simulink model "dynmodel_KUKA"  (R2016a)
settings: Solver=VariableStepAuto  StartTime=0.0  StopTime=10.0  MaxStep=1e-3  RelTol=1e-3
values from neighbouring files (symbols this model uses):
  th_DHM = -th_KUKA + offset    [dynamique_youbot.m]
libraries: simulink x1, dspmtrx3 x1
settings Model: Creator=Makarov_Mar  LastModifiedBy=Makarov_Mar

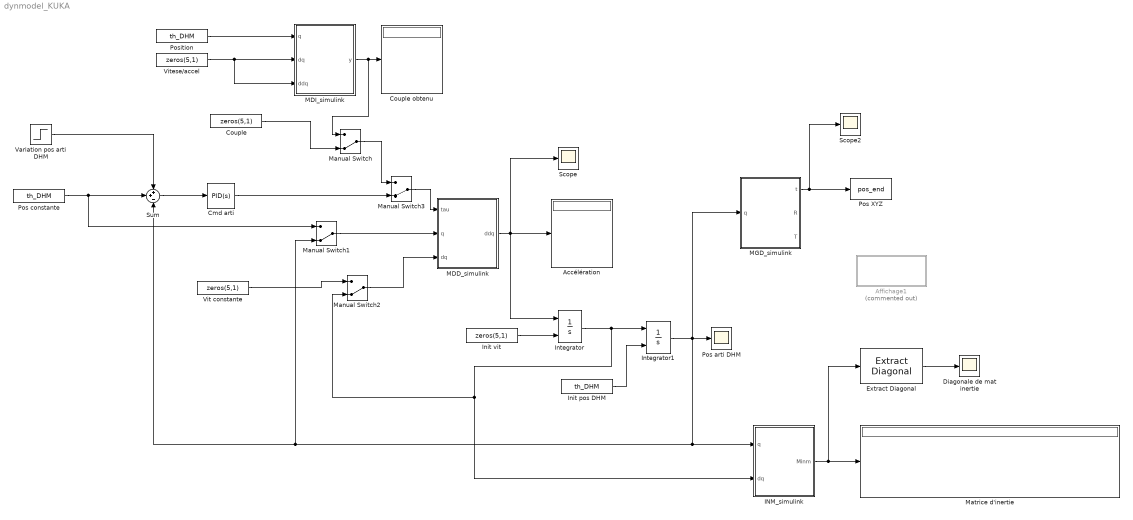
== system dynmodel_KUKA ==
  Accélération : Display
  Affichage1 : Subsystem  Commented=on  StopFcn=|
      | tps_sim =  pos_end.time;
      | PendX = pos_end.signals.values(:,1);
      | PendY = pos_end.signals.values(:,2);
      | PendZ = pos_end.signals.values(:,3);
      | 
      | figure(20)
      | for k = 1:70:length(tps_sim)
      |   figure(20)
      |   plot3(0,0,0,'r.','markersize',20); grid on; hold on
      |   axis([-0.7 0.7 -0.7 0.7 -1 +1])
      |   plot3(PendX(k),PendY(k),PendZ(k),'b.','markersize',10)
      |   xlabel('xB'); ylabel('yB'); zlabel('zB')
      |   title('xend : vert, yend : cyan, zend : rouge') 
      |   pause(0.1)
      | end
  Cmd arti : simulink/Continuous/PID Controller  Controller=PID  TimeDomain=Continuous-time  SampleTime=-1  IntegratorMethod=Forward Euler  FilterMethod=Forward Euler  Form=Parallel  UseFilter=on  ControllerParametersSource=internal  P=Kp.'  I=zeros(5,1)  D=Kd.'  N=10  InitialConditionSource=internal  InitialConditionForIntegrator=0  InitialConditionForFilter=0  ExternalReset=none  LimitOutput=off  UpperSaturationLimit=inf  LowerSaturationLimit=-inf  LinearizeAsGain=on  AntiWindupMode=none  Kb=1  TrackingMode=off  Kt=1  PParamMin=[]  PParamMax=[]  IParamMin=[]  IParamMax=[]  DParamMin=[]  DParamMax=[]  NParamMin=[]  NParamMax=[]  KbParamMin=[]  KbParamMax=[]  KtParamMin=[]  KtParamMax=[]  POutMin=[]  POutMax=[]  IOutMin=[]  IOutMax=[]  DOutMin=[]  DOutMax=[]  NOutMin=[]  NOutMax=[]  KbOutMin=[]  KbOutMax=[]  KtOutMin=[]  KtOutMax=[]  IntegratorOutMin=[]  IntegratorOutMax=[]  FilterOutMin=[]  FilterOutMax=[]  SumOutMin=[]  SumOutMax=[]  SumI1OutMin=[]  SumI1OutMax=[]  SumI2OutMin=[]  SumI2OutMax=[]  SumI3OutMin=[]  SumI3OutMax=[]  SumDOutMin=[]  SumDOutMax=[]  SaturationOutMin=[]  SaturationOutMax=[]  IntegratorContinuousStateAttributes=''  IntegratorStateMustResolveToSignalObject=off  IntegratorRTWStateStorageClass=Auto  FilterContinuousStateAttributes=''  FilterStateMustResolveToSignalObject=off  FilterRTWStateStorageClass=Auto  DifferentiatorICPrevScaledInput=0  DifferentiatorOutMin=[]  DifferentiatorOutMax=[]
  Couple : Constant  Value=zeros(5,1)  VectorParams1D=off
  Couple obtenu : Display
  Diagonale de mat inertie : Scope
  Extract Diagonal : dspmtrx3/Extract Diagonal
  INM_simulink : MATLAB Function  TreatAsAtomicUnit=on
  Init pos DHM : Constant  Value=th_DHM  VectorParams1D=off
  Init vit : Constant  Value=zeros(5,1)  VectorParams1D=off
  Integrator : Integrator  InitialConditionSource=external
  Integrator1 : Integrator  InitialConditionSource=external
  MDD_simulink : MATLAB Function  TreatAsAtomicUnit=on
  MDI_simulink : MATLAB Function  TreatAsAtomicUnit=on
  MGD_simulink : MATLAB Function  TreatAsAtomicUnit=on
  Manual Switch{,1..3} (4 alike) : ManualSwitch  CurrentSetting=0
  Matrice d'inertie : Display
  Pos XYZ : ToWorkspace  VariableName=pos_end  SaveFormat=Structure With Time  SampleTime=-1
  Pos arti DHM : Scope
  Pos constante : Constant  Value=th_DHM  VectorParams1D=off
  Position : Constant  Value=th_DHM  VectorParams1D=off
  Scope : Scope
  Scope2 : Scope
  Sum : Sum  Inputs=++-
  Variation pos arti DHM : Step  After=[0 pi/2 0 0 0]  SampleTime=0
  Vit constante : Constant  Value=zeros(5,1)  VectorParams1D=off
  Vitese/accel : Constant  Value=zeros(5,1)  VectorParams1D=off
  wires:
  Vitese/accel/1 -> MDI_simulink/2(dq), MDI_simulink/3(ddq)
  Position/1 -> MDI_simulink/1(q)
  MDI_simulink/1(y) -> Manual Switch/1, Couple obtenu/1
  MDD_simulink/1(ddq) -> Integrator/1, Scope/1, Accélération/1
  Couple/1 -> Manual Switch/2
  Integrator/1 -> INM_simulink/2(dq), Manual Switch2/2, Integrator1/1
  Init vit/1 -> Integrator/2
  Init pos DHM/1 -> Integrator1/2
  Pos constante/1 -> Sum/2, Manual Switch1/1
  Manual Switch1/1 -> MDD_simulink/2(q)
  Vit constante/1 -> Manual Switch2/1
  Manual Switch2/1 -> MDD_simulink/3(dq)
  Integrator1/1 -> MGD_simulink/1(q), Sum/3, Manual Switch1/2, INM_simulink/1(q), Pos arti DHM/1
  MGD_simulink/1(t) -> Scope2/1, Pos XYZ/1
  INM_simulink/1(Minm) -> Extract Diagonal/1, Matrice d'inertie/1
  Extract Diagonal/1 -> Diagonale de mat inertie/1
  Manual Switch/1 -> Manual Switch3/1
  Manual Switch3/1 -> MDD_simulink/1(tau)
  Cmd arti/1 -> Manual Switch3/2
  Sum/1 -> Cmd arti/1
  Variation pos arti DHM/1 -> Sum/1

== system dynmodel_KUKA/Affichage1 ==

== matlab function dynmodel_KUKA/MDD_simulink ==
  data: tau input; q input; dq input; ddq output size=5; param parameter
function ddq = fcn(tau,q,dq, param)

th1 = q(1);
th2 = q(2);
th3 = q(3);
th4 = q(4);
th5 = q(5);

QP1 = dq(1);
QP2 = dq(2);
QP3 = dq(3);
QP4 = dq(4);
QP5 = dq(5);

GAM1 =tau(1);
GAM2 =tau(2);
GAM3 =tau(3);
GAM4 =tau(4);
GAM5 = tau(5);

% introduction des paramètres
GZ=param.GZ;
XXR2=param.XXR2;
XXR3=param.XXR3;
XXR4=param.XXR4;
XXR5=param.XXR5;
XY2=param.XY2;
XY3=param.XY3;
XY4=param.XY4;
XY5=param.XY5;
XZR2=param.XZR2;
XZR3=param.XZR3;
XZ4=param.XZ4;
XZ5=param.XZ5;
YZ2=param.YZ2;
YZ3=param.YZ3;
YZ4=param.YZ4;
YZ5=param.YZ5;
ZZR1=param.ZZR1;
ZZR2=param.ZZR2;
ZZR3=param.ZZR3;
ZZR4=param.ZZR4;
ZZ5=param.ZZ5;
MXR2=param.MXR2;
MXR3=param.MXR3;
MX4=param.MX4;
MX5=param.MX5;
MY2=param.MY2;
MY3=param.MY3;
MYR4=param.MYR4;
MY5=param.MY5;
IA3=param.IA3;
IA4=param.IA4;
IA5=param.IA5;
FV1=param.FV1;
FV2=param.FV2;
FV3=param.FV3;
FV4=param.FV4;
FV5=param.FV5;
FS1=param.FS1;
FS2=param.FS2;
FS3=param.FS3;
FS4=param.FS4;
FS5=param.FS5;
d1=param.d1;
r1=param.r1;
d2=param.d2;
d3=param.d3;
d4=param.d4;

FX5=0;
FY5=0;
FZ5=0;
CX5=0;
CY5=0;
CZ5=0;

% code généré OpenSymoro
C1 = cos(th1);
S1 = sin(th1);
C2 = cos(th2);
S2 = sin(th2);
C3 = cos(th3);
S3 = sin(th3);
C4 = cos(th4);
S4 = sin(th4);
C5 = cos(th5);
S5 = sin(th5);
WI12 = QP1*S2;
WI22 = C2*QP1;
WQ12 = QP2*WI22;
WQ22 = -QP2*WI12;
LW12 = -C2*QP1^2*d2;
LW22 = QP1^2*S2*d2;
JW12 = QP2*XZR2 + WI12*XXR2 + WI22*XY2;
JW22 = QP2*YZ2 + WI12*XY2;
JW32 = QP2*ZZR2 + WI12*XZR2 + WI22*YZ2;
KW12 = -JW22*QP2 + JW32*WI22;
KW22 = JW12*QP2 - JW32*WI12;
KW32 = -JW12*WI22 + JW22*WI12;
SW12 = -MXR2*QP2^2 + WI22*(-MXR2*WI22 + MY2*WI12);
SW22 = -MY2*QP2^2 - WI12*(-MXR2*WI22 + MY2*WI12);
SW32 = MXR2*QP2*WI12 + MY2*QP2*WI22;
WI13 = C3*WI12 + S3*WI22;
WI23 = C3*WI22 - S3*WI12;
W33 = QP2 + QP3;
JPR133 = S3*d3;
JPR233 = C3*d3;
WQ13 = QP3*WI23;
WQ23 = -QP3*WI13;
LW13 = C3*(-QP2^2*d3 - WI22^2*d3) + S3*WI12*WI22*d3;
LW23 = C3*WI12*WI22*d3 - S3*(-QP2^2*d3 - WI22^2*d3);
LW33 = QP2*WI12*d3;
JW13 = W33*XZR3 + WI13*XXR3 + WI23*XY3;
JW23 = W33*YZ3 + WI13*XY3;
JW33 = W33*ZZR3 + WI13*XZR3 + WI23*YZ3;
KW13 = -JW23*W33 + JW33*WI23;
KW23 = JW13*W33 - JW33*WI13;
KW33 = -JW13*WI23 + JW23*WI13;
SW13 = -MXR3*W33^2 + WI23*(-MXR3*WI23 + MY3*WI13);
SW23 = -MY3*W33^2 - WI13*(-MXR3*WI23 + MY3*WI13);
SW33 = MXR3*W33*WI13 + MY3*W33*WI23;
WI14 = C4*WI13 + S4*WI23;
WI24 = C4*WI23 - S4*WI13;
W34 = QP4 + W33;
JPR134 = S4*d4;
JPR234 = C4*d4;
WQ14 = QP4*WI24;
WQ24 = -QP4*WI14;
LW14 = C4*(-W33^2*d4 - WI23^2*d4) + S4*WI13*WI23*d4;
LW24 = C4*WI13*WI23*d4 - S4*(-W33^2*d4 - WI23^2*d4);
LW34 = W33*WI13*d4;
JW14 = W34*XZ4 + WI14*XXR4 + WI24*XY4;
JW24 = W34*YZ4 + WI14*XY4;
JW34 = W34*ZZR4 + WI14*XZ4 + WI24*YZ4;
KW14 = -JW24*W34 + JW34*WI24;
KW24 = JW14*W34 - JW34*WI14;
KW34 = -JW14*WI24 + JW24*WI14;
SW14 = -MX4*W34^2 + WI24*(-MX4*WI24 + MYR4*WI14);
SW24 = -MYR4*W34^2 - WI14*(-MX4*WI24 + MYR4*WI14);
SW34 = MX4*W34*WI14 + MYR4*W34*WI24;
WI15 = C5*WI14 - S5*W34;
WI25 = -C5*W34 - S5*WI14;
W35 = QP5 + WI24;
WQ15 = QP5*WI25;
WQ25 = -QP5*WI15;
JW15 = W35*XZ5 + WI15*XXR5 + WI25*XY5;
JW25 = W35*YZ5 + WI15*XY5;
JW35 = W35*ZZ5 + WI15*XZ5 + WI25*YZ5;
KW15 = -JW25*W35 + JW35*WI25;
KW25 = JW15*W35 - JW35*WI15;
KW35 = -JW15*WI25 + JW25*WI15;
SW15 = -MX5*W35^2 + WI25*(-MX5*WI25 + MY5*WI15);
SW25 = -MY5*W35^2 - WI15*(-MX5*WI25 + MY5*WI15);
SW35 = MX5*W35*WI15 + MY5*W35*WI25;
BETA15 = -FX5 - SW15;
BETA25 = -FY5 - SW25;
BETA35 = -FZ5 - SW35;
BETA45 = -CX5 - KW15;
BETA55 = -CY5 - KW25;
BETA65 = -CZ5 - KW35;
GW5 = BETA65 - FS5*sign(QP5) - FV5*QP5 + GAM5;
JD5 = 1/(IA5 + ZZ5);
JU15 = -JD5*MY5;
JU25 = JD5*MX5;
JU45 = JD5*XZ5;
JU55 = JD5*YZ5;
JU65 = JD5*ZZ5;
GK115 = JU15*MY5;
GK215 = JU25*MY5;
GK415 = JU45*MY5;
GK515 = JU55*MY5;
GK615 = JU65*MY5 - MY5;
GK125 = -JU15*MX5;
GK225 = -JU25*MX5;
GK425 = -JU45*MX5;
GK525 = -JU55*MX5;
GK625 = -JU65*MX5 + MX5;
GK145 = -JU15*XZ5;
GK245 = -JU25*XZ5;
GK445 = -JU45*XZ5 + XXR5;
GK545 = -JU55*XZ5 + XY5;
GK645 = -JU65*XZ5 + XZ5;
GK155 = -JU15*YZ5;
GK255 = -JU25*YZ5;
GK455 = -JU45*YZ5 + XY5;
GK555 = -JU55*YZ5;
GK655 = -JU65*YZ5 + YZ5;
GK465 = -JU45*ZZ5 + XZ5;
GK565 = -JU55*ZZ5 + YZ5;
GK665 = -JU65*ZZ5 + ZZ5;
NG15 = GK145*WQ15 + GK155*WQ25;
NG25 = GK245*WQ15 + GK255*WQ25;
NG35 = -MX5*WQ25 + MY5*WQ15;
NG45 = GK445*WQ15 + GK455*WQ25;
NG55 = GK545*WQ15 + GK555*WQ25;
NG65 = GK645*WQ15 + GK655*WQ25;
VS15 = GW5*JU15 + NG15;
VS25 = GW5*JU25 + NG25;
VS45 = GW5*JU45 + NG45;
VS55 = GW5*JU55 + NG55;
VS65 = GW5*JU65 + NG65;
AP15 = -BETA15 + VS15;
AP25 = -BETA25 + VS25;
AP35 = -BETA35 + NG35;
AP45 = -BETA45 + VS45;
AP55 = -BETA55 + VS55;
AP65 = -BETA65 + VS65;
GX115 = C5*GK115 - GK215*S5;
GX315 = -C5*GK215 - GK115*S5;
GX415 = C5*GK415 - GK515*S5;
GX615 = -C5*GK515 - GK415*S5;
GX125 = C5*GK125 - GK225*S5;
GX325 = -C5*GK225 - GK125*S5;
GX425 = C5*GK425 - GK525*S5;
GX625 = -C5*GK525 - GK425*S5;
GX435 = C5*MY5 + MX5*S5;
GX635 = C5*MX5 - MY5*S5;
GX445 = C5*GK445 - GK545*S5;
GX645 = -C5*GK545 - GK445*S5;
GX455 = C5*GK455 - GK555*S5;
GX655 = -C5*GK555 - GK455*S5;
GX665 = -C5*GK565 - GK465*S5;
TKT115 = C5*GX115 - GX125*S5;
TKT315 = C5*GX315 - GX325*S5;
TKT415 = C5*GX415 - GX425*S5;
TKT515 = C5*GK615 - GK625*S5;
TKT615 = C5*GX615 - GX625*S5;
TKT335 = -C5*GX325 - GX315*S5;
TKT435 = -C5*GX425 - GX415*S5;
TKT535 = -C5*GK625 - GK615*S5;
TKT635 = -C5*GX625 - GX615*S5;
TKT445 = C5*GX445 - GX455*S5;
TKT545 = C5*GK645 - GK655*S5;
TKT645 = C5*GX645 - GX655*S5;
TKT665 = -C5*GX655 - GX645*S5;
ALJI15 = AP15*C5 - AP25*S5;
ALJI35 = -AP15*S5 - AP25*C5;
ALJI45 = AP45*C5 - AP55*S5;
ALJI65 = -AP45*S5 - AP55*C5;
MJE614 = -MYR4 + TKT615;
MJE624 = GX635 + MX4;
MJE434 = MYR4 + TKT435;
MJE534 = -MX4 + TKT535;
MJE444 = TKT445 + XXR4;
MJE544 = TKT545 + XY4;
MJE644 = TKT645 + XZ4;
MJE654 = GX665 + YZ4;
MJE664 = TKT665 + ZZR4;
VBE14 = -ALJI15 - SW14;
VBE24 = -AP35 - SW24;
VBE34 = -ALJI35 - SW34;
VBE44 = -ALJI45 - KW14;
VBE54 = -AP65 - KW24;
VBE64 = -ALJI65 - KW34;
GW4 = -FS4*sign(QP4) - FV4*QP4 + GAM4 + VBE64;
JD4 = 1/(IA4 + MJE664);
JU14 = JD4*MJE614;
JU24 = JD4*MJE624;
JU34 = JD4*TKT635;
JU44 = JD4*MJE644;
JU54 = JD4*MJE654;
JU64 = JD4*MJE664;
GK114 = -JU14*MJE614 + TKT115;
GK214 = -JU24*MJE614;
GK314 = -JU34*MJE614 + TKT315;
GK414 = -JU44*MJE614 + TKT415;
GK514 = -JU54*MJE614 + TKT515;
GK614 = -JU64*MJE614 + MJE614;
GK124 = -JU14*MJE624;
GK224 = -JU24*MJE624;
GK324 = -JU34*MJE624;
GK424 = GX435 - JU44*MJE624;
GK524 = -JU54*MJE624;
GK624 = -JU64*MJE624 + MJE624;
GK134 = -JU14*TKT635 + TKT315;
GK234 = -JU24*TKT635;
GK334 = -JU34*TKT635 + TKT335;
GK434 = -JU44*TKT635 + MJE434;
GK534 = -JU54*TKT635 + MJE534;
GK634 = -JU64*TKT635 + TKT635;
GK144 = -JU14*MJE644 + TKT415;
GK244 = GX435 - JU24*MJE644;
GK344 = -JU34*MJE644 + MJE434;
GK444 = -JU44*MJE644 + MJE444;
GK544 = -JU54*MJE644 + MJE544;
GK644 = -JU64*MJE644 + MJE644;
GK154 = -JU14*MJE654 + TKT515;
GK254 = -JU24*MJE654;
GK354 = -JU34*MJE654 + MJE534;
GK454 = -JU44*MJE654 + MJE544;
GK554 = GK665 - JU54*MJE654;
GK654 = -JU64*MJE654 + MJE654;
GK164 = -JU14*MJE664 + MJE614;
GK264 = -JU24*MJE664 + MJE624;
GK664 = -JU64*MJE664 + MJE664;
NG14 = GK114*LW14 + GK124*LW24 + GK134*LW34 + GK144*WQ14 + GK154*WQ24;
NG24 = GK214*LW14 + GK224*LW24 + GK234*LW34 + GK244*WQ14 + GK254*WQ24;
NG34 = GK314*LW14 + GK324*LW24 + GK334*LW34 + GK344*WQ14 + GK354*WQ24;
NG44 = GK414*LW14 + GK424*LW24 + GK434*LW34 + GK444*WQ14 + GK454*WQ24;
NG54 = GK514*LW14 + GK524*LW24 + GK534*LW34 + GK544*WQ14 + GK554*WQ24;
NG64 = GK614*LW14 + GK624*LW24 + GK634*LW34 + GK644*WQ14 + GK654*WQ24;
VS14 = GW4*JU14 + NG14;
VS24 = GW4*JU24 + NG24;
VS34 = GW4*JU34 + NG34;
VS44 = GW4*JU44 + NG44;
VS54 = GW4*JU54 + NG54;
VS64 = GW4*JU64 + NG64;
AP14 = -VBE14 + VS14;
AP24 = -VBE24 + VS24;
AP34 = -VBE34 + VS34;
AP44 = -VBE44 + VS44;
AP54 = -VBE54 + VS54;
AP64 = -VBE64 + VS64;
GX114 = C4*GK114 - GK214*S4;
GX214 = C4*GK214 + GK114*S4;
GX414 = C4*GK414 - GK514*S4;
GX514 = C4*GK514 - GK314*d4 + GK414*S4;
GX614 = GK114*JPR134 + GK214*JPR234 + GK614;
GX124 = C4*GK124 - GK224*S4;
GX224 = C4*GK224 + GK124*S4;
GX424 = C4*GK424 - GK524*S4;
GX524 = C4*GK524 - GK324*d4 + GK424*S4;
GX624 = GK124*JPR134 + GK224*JPR234 + GK624;
GX434 = C4*GK434 - GK534*S4;
GX534 = C4*GK534 - GK334*d4 + GK434*S4;
GX634 = GK134*JPR134 + GK234*JPR234 + GK634;
GX444 = C4*GK444 - GK544*S4;
GX544 = C4*GK544 - GK344*d4 + GK444*S4;
GX644 = GK144*JPR134 + GK244*JPR234 + GK644;
GX454 = C4*GK454 - GK554*S4;
GX554 = C4*GK554 - GK354*d4 + GK454*S4;
GX654 = GK154*JPR134 + GK254*JPR234 + GK654;
GX664 = GK164*JPR134 + GK264*JPR234 + GK664;
TKT114 = C4*GX114 - GX124*S4;
TKT214 = C4*GX214 - GX224*S4;
TKT314 = C4*GK314 - GK324*S4;
TKT414 = C4*GX414 - GX424*S4;
TKT514 = C4*GX514 - GX524*S4;
TKT614 = C4*GX614 - GX624*S4;
TKT224 = C4*GX224 + GX214*S4;
TKT324 = C4*GK324 + GK314*S4;
TKT424 = C4*GX424 + GX414*S4;
TKT524 = C4*GX524 + GX514*S4;
TKT624 = C4*GX624 + GX614*S4;
TKT444 = C4*GX444 - GX454*S4;
TKT544 = C4*GX544 - GX554*S4;
TKT644 = C4*GX644 - GX654*S4;
TKT554 = C4*GX554 - GX534*d4 + GX544*S4;
TKT654 = C4*GX654 - GX634*d4 + GX644*S4;
TKT664 = GX614*JPR134 + GX624*JPR234 + GX664;
ALJI14 = AP14*C4 - AP24*S4;
ALJI24 = AP14*S4 + AP24*C4;
ALJI44 = AP44*C4 - AP54*S4;
ALJI54 = -AP34*d4 + AP44*S4 + AP54*C4;
ALJI64 = AP14*JPR134 + AP24*JPR234 + AP64;
MJE613 = -MY3 + TKT614;
MJE623 = MXR3 + TKT624;
MJE433 = GX434 + MY3;
MJE533 = GX534 - MXR3;
MJE443 = TKT444 + XXR3;
MJE543 = TKT544 + XY3;
MJE643 = TKT644 + XZR3;
MJE653 = TKT654 + YZ3;
MJE663 = TKT664 + ZZR3;
VBE13 = -ALJI14 - SW13;
VBE23 = -ALJI24 - SW23;
VBE33 = -AP34 - SW33;
VBE43 = -ALJI44 - KW13;
VBE53 = -ALJI54 - KW23;
VBE63 = -ALJI64 - KW33;
GW3 = -FS3*sign(QP3) - FV3*QP3 + GAM3 + VBE63;
JD3 = 1/(IA3 + MJE663);
JU13 = JD3*MJE613;
JU23 = JD3*MJE623;
JU33 = GX634*JD3;
JU43 = JD3*MJE643;
JU53 = JD3*MJE653;
JU63 = JD3*MJE663;
GK113 = -JU13*MJE613 + TKT114;
GK213 = -JU23*MJE613 + TKT214;
GK313 = -JU33*MJE613 + TKT314;
GK413 = -JU43*MJE613 + TKT414;
GK513 = -JU53*MJE613 + TKT514;
GK613 = -JU63*MJE613 + MJE613;
GK123 = -JU13*MJE623 + TKT214;
GK223 = -JU23*MJE623 + TKT224;
GK323 = -JU33*MJE623 + TKT324;
GK423 = -JU43*MJE623 + TKT424;
GK523 = -JU53*MJE623 + TKT524;
GK623 = -JU63*MJE623 + MJE623;
GK133 = -GX634*JU13 + TKT314;
GK233 = -GX634*JU23 + TKT324;
GK333 = GK334 - GX634*JU33;
GK433 = -GX634*JU43 + MJE433;
GK533 = -GX634*JU53 + MJE533;
GK633 = -GX634*JU63 + GX634;
GK143 = -JU13*MJE643 + TKT414;
GK243 = -JU23*MJE643 + TKT424;
GK343 = -JU33*MJE643 + MJE433;
GK443 = -JU43*MJE643 + MJE443;
GK543 = -JU53*MJE643 + MJE543;
GK643 = -JU63*MJE643 + MJE643;
GK153 = -JU13*MJE653 + TKT514;
GK253 = -JU23*MJE653 + TKT524;
GK353 = -JU33*MJE653 + MJE533;
GK453 = -JU43*MJE653 + MJE543;
GK553 = -JU53*MJE653 + TKT554;
GK653 = -JU63*MJE653 + MJE653;
GK163 = -JU13*MJE663 + MJE613;
GK263 = -JU23*MJE663 + MJE623;
GK663 = -JU63*MJE663 + MJE663;
NG13 = GK113*LW13 + GK123*LW23 + GK133*LW33 + GK143*WQ13 + GK153*WQ23;
NG23 = GK213*LW13 + GK223*LW23 + GK233*LW33 + GK243*WQ13 + GK253*WQ23;
NG33 = GK313*LW13 + GK323*LW23 + GK333*LW33 + GK343*WQ13 + GK353*WQ23;
NG43 = GK413*LW13 + GK423*LW23 + GK433*LW33 + GK443*WQ13 + GK453*WQ23;
NG53 = GK513*LW13 + GK523*LW23 + GK533*LW33 + GK543*WQ13 + GK553*WQ23;
NG63 = GK613*LW13 + GK623*LW23 + GK633*LW33 + GK643*WQ13 + GK653*WQ23;
VS13 = GW3*JU13 + NG13;
VS23 = GW3*JU23 + NG23;
VS33 = GW3*JU33 + NG33;
VS43 = GW3*JU43 + NG43;
VS53 = GW3*JU53 + NG53;
VS63 = GW3*JU63 + NG63;
AP13 = -VBE13 + VS13;
AP23 = -VBE23 + VS23;
AP33 = -VBE33 + VS33;
AP43 = -VBE43 + VS43;
AP53 = -VBE53 + VS53;
AP63 = -VBE63 + VS63;
GX413 = C3*GK413 - GK513*S3;
GX513 = C3*GK513 - GK313*d3 + GK413*S3;
GX613 = GK113*JPR133 + GK213*JPR233 + GK613;
GX423 = C3*GK423 - GK523*S3;
GX523 = C3*GK523 - GK323*d3 + GK423*S3;
GX623 = GK123*JPR133 + GK223*JPR233 + GK623;
GX433 = C3*GK433 - GK533*S3;
GX533 = C3*GK533 - GK333*d3 + GK433*S3;
GX633 = GK133*JPR133 + GK233*JPR233 + GK633;
GX443 = C3*GK443 - GK543*S3;
GX543 = C3*GK543 - GK343*d3 + GK443*S3;
GX643 = GK143*JPR133 + GK243*JPR233 + GK643;
GX453 = C3*GK453 - GK553*S3;
GX553 = C3*GK553 - GK353*d3 + GK453*S3;
GX653 = GK153*JPR133 + GK253*JPR233 + GK653;
GX663 = GK163*JPR133 + GK263*JPR233 + GK663;
TKT313 = C3*GK313 - GK323*S3;
TKT413 = C3*GX413 - GX423*S3;
TKT513 = C3*GX513 - GX523*S3;
TKT613 = C3*GX613 - GX623*S3;
TKT323 = C3*GK323 + GK313*S3;
TKT423 = C3*GX423 + GX413*S3;
TKT523 = C3*GX523 + GX513*S3;
TKT623 = C3*GX623 + GX613*S3;
TKT443 = C3*GX443 - GX453*S3;
TKT543 = C3*GX543 - GX553*S3;
TKT643 = C3*GX643 - GX653*S3;
TKT553 = C3*GX553 - GX533*d3 + GX543*S3;
TKT653 = C3*GX653 - GX633*d3 + GX643*S3;
TKT663 = GX613*JPR133 + GX623*JPR233 + GX663;
ALJI43 = AP43*C3 - AP53*S3;
ALJI53 = -AP33*d3 + AP43*S3 + AP53*C3;
ALJI63 = AP13*JPR133 + AP23*JPR233 + AP63;
MJE612 = -MY2 + TKT613;
MJE622 = MXR2 + TKT623;
MJE432 = GX433 + MY2;
MJE532 = GX533 - MXR2;
MJE442 = TKT443 + XXR2;
MJE542 = TKT543 + XY2;
MJE642 = TKT643 + XZR2;
MJE652 = TKT653 + YZ2;
MJE662 = TKT663 + ZZR2;
VBE32 = -AP33 - SW32;
VBE42 = -ALJI43 - KW12;
VBE52 = -ALJI53 - KW22;
VBE62 = -ALJI63 - KW32;
GW2 = -FS2*sign(QP2) - FV2*QP2 + GAM2 + VBE62;
JD2 = 1/MJE662;
JU12 = JD2*MJE612;
JU22 = JD2*MJE622;
JU32 = GX633*JD2;
JU42 = JD2*MJE642;
JU52 = JD2*MJE652;
GK312 = -JU32*MJE612 + TKT313;
GK412 = -JU42*MJE612 + TKT413;
GK512 = -JU52*MJE612 + TKT513;
GK322 = -JU32*MJE622 + TKT323;
GK422 = -JU42*MJE622 + TKT423;
GK522 = -JU52*MJE622 + TKT523;
GK332 = GK333 - GX633*JU32;
GK432 = -GX633*JU42 + MJE432;
GK532 = -GX633*JU52 + MJE532;
GK342 = -JU32*MJE642 + MJE432;
GK442 = -JU42*MJE642 + MJE442;
GK542 = -JU52*MJE642 + MJE542;
GK352 = -JU32*MJE652 + MJE532;
GK452 = -JU42*MJE652 + MJE542;
GK552 = -JU52*MJE652 + TKT553;
NG32 = GK312*LW12 + GK322*LW22 + GK342*WQ12 + GK352*WQ22;
NG42 = GK412*LW12 + GK422*LW22 + GK442*WQ12 + GK452*WQ22;
NG52 = GK512*LW12 + GK522*LW22 + GK542*WQ12 + GK552*WQ22;
VS32 = GW2*JU32 + NG32;
VS42 = GW2*JU42 + NG42;
VS52 = GW2*JU52 + NG52;
AP32 = -VBE32 + VS32;
AP42 = -VBE42 + VS42;
AP52 = -VBE52 + VS52;
GX612 = C2*GK512 - GK312*d2 + GK412*S2;
GX622 = C2*GK522 - GK322*d2 + GK422*S2;
GX632 = C2*GK532 - GK332*d2 + GK432*S2;
GX642 = C2*GK542 - GK342*d2 + GK442*S2;
GX652 = C2*GK552 - GK352*d2 + GK452*S2;
TKT632 = C2*GX622 + GX612*S2;
TKT662 = C2*GX652 - GX632*d2 + GX642*S2;
ALJI62 = -AP32*d2 + AP42*S2 + AP52*C2;
MJE661 = TKT662 + ZZR1;
GW1 = -ALJI62 - FS1*sign(QP1) - FV1*QP1 + GAM1;
JD1 = 1/MJE661;
JU31 = JD1*TKT632;
GU1 = -GZ*JU31;
QDP1 = -GU1 + GW1*JD1;


VR12 = -GZ*S2 + LW12;
VR22 = -C2*GZ + LW22;
VR32 = -QDP1*d2;
VR42 = QDP1*S2 + WQ12;
VR52 = C2*QDP1 + WQ22;
GU2 = JU12*VR12 + JU22*VR22 + JU32*VR32 + JU42*VR42 + JU52*VR52;
QDP2 = -GU2 + GW2*JD2;


VR13 = C3*VR12 + JPR133*QDP2 + LW13 + S3*VR22;
VR23 = C3*VR22 + JPR233*QDP2 + LW23 - S3*VR12;
VR33 = LW33 + VR32 - VR52*d3;
VR43 = C3*VR42 + S3*VR52 + WQ13;
VR53 = C3*VR52 - S3*VR42 + WQ23;
GU3 = JU13*VR13 + JU23*VR23 + JU33*VR33 + JU43*VR43 + JU53*VR53 + JU63*QDP2;
QDP3 = -GU3 + GW3*JD3;

WP33 = QDP2 + QDP3;
VR14 = C4*VR13 + JPR134*WP33 + LW14 + S4*VR23;
VR24 = C4*VR23 + JPR234*WP33 + LW24 - S4*VR13;
VR34 = LW34 + VR33 - VR53*d4;
VR44 = C4*VR43 + S4*VR53 + WQ14;
VR54 = C4*VR53 - S4*VR43 + WQ24;
GU4 = JU14*VR14 + JU24*VR24 + JU34*VR34 + JU44*VR44 + JU54*VR54 + JU64*WP33;
QDP4 = -GU4 + GW4*JD4;

WP34 = QDP4 + WP33;
VR15 = C5*VR14 - S5*VR34;
VR25 = -C5*VR34 - S5*VR14;
VR45 = C5*VR44 - S5*WP34 + WQ15;
VR55 = -C5*WP34 - S5*VR44 + WQ25;
GU5 = JU15*VR15 + JU25*VR25 + JU45*VR45 + JU55*VR55 + JU65*VR54;
QDP5 = -GU5 + GW5*JD5;

ddq = [QDP1 QDP2 QDP3 QDP4 QDP5].';

== matlab function dynmodel_KUKA/MDI_simulink ==
  data: q input; dq input; ddq input; y output size=5; param parameter
function y = fcn(q,dq, ddq, param)

th2 = q(2);
th3 = q(3);
th4 = q(4);
th5 = q(5);

QP1 = dq(1);
QP2 = dq(2);
QP3 = dq(3);
QP4 = dq(4);
QP5 = dq(5);

QDP1 = ddq(1);
QDP2 = ddq(2);
QDP3 = ddq(3);
QDP4 = ddq(4);
QDP5 = ddq(5);

% introduction des paramètres
GZ=param.GZ;
XXR2=param.XXR2;
XXR3=param.XXR3;
XXR4=param.XXR4;
XXR5=param.XXR5;
XY2=param.XY2;
XY3=param.XY3;
XY4=param.XY4;
XY5=param.XY5;
XZR2=param.XZR2;
XZR3=param.XZR3;
XZ4=param.XZ4;
XZ5=param.XZ5;
YZ2=param.YZ2;
YZ3=param.YZ3;
YZ4=param.YZ4;
YZ5=param.YZ5;
ZZR1=param.ZZR1;
ZZR2=param.ZZR2;
ZZR3=param.ZZR3;
ZZR4=param.ZZR4;
ZZ5=param.ZZ5;
MXR2=param.MXR2;
MXR3=param.MXR3;
MX4=param.MX4;
MX5=param.MX5;
MY2=param.MY2;
MY3=param.MY3;
MYR4=param.MYR4;
MY5=param.MY5;
IA3=param.IA3;
IA4=param.IA4;
IA5=param.IA5;
FV1=param.FV1;
FV2=param.FV2;
FV3=param.FV3;
FV4=param.FV4;
FV5=param.FV5;
FS1=param.FS1;
FS2=param.FS2;
FS3=param.FS3;
FS4=param.FS4;
FS5=param.FS5;
d1=param.d1;
r1=param.r1;
d2=param.d2;
d3=param.d3;
d4=param.d4;

FX5=0;
FY5=0;
FZ5=0;
CX5=0;
CY5=0;
CZ5=0;

% code généré OpenSymoro
C2 = cos(th2);
S2 = sin(th2);
C3 = cos(th3);
S3 = sin(th3);
C4 = cos(th4);
S4 = sin(th4);
C5 = cos(th5);
S5 = sin(th5);
DV61 = QP1^2;
W12 = QP1*S2;
W22 = C2*QP1;
WP12 = QDP1*S2 + QP2*W22;
WP22 = C2*QDP1 - QP2*W12;
DV22 = W12*W22;
DV32 = QP2*W12;
DV42 = W22^2;
DV52 = QP2*W22;
DV62 = QP2^2;
U112 = -DV42 - DV62;
U212 = DV22 + QDP2;
U312 = DV32 - WP22;
U322 = DV52 + WP12;
VSP12 = -DV61*d2;
VSP22 = QDP1*d2;
VP12 = C2*VSP12 - GZ*S2;
VP22 = -C2*GZ - S2*VSP12;
W13 = C3*W12 + S3*W22;
W23 = C3*W22 - S3*W12;
W33 = QP2 + QP3;
WP13 = C3*WP12 + QP3*W23 + S3*WP22;
WP23 = C3*WP22 - QP3*W13 - S3*WP12;
WP33 = QDP2 + QDP3;
DV13 = W13^2;
DV23 = W13*W23;
DV33 = W13*W33;
DV43 = W23^2;
DV53 = W23*W33;
DV63 = W33^2;
U113 = -DV43 - DV63;
U213 = DV23 + WP33;
U313 = DV33 - WP23;
U123 = DV23 - WP33;
U223 = -DV13 - DV63;
U323 = DV53 + WP13;
VSP13 = U112*d3 + VP12;
VSP23 = U212*d3 + VP22;
VSP33 = U312*d3 - VSP22;
VP13 = C3*VSP13 + S3*VSP23;
VP23 = C3*VSP23 - S3*VSP13;
W14 = C4*W13 + S4*W23;
W24 = C4*W23 - S4*W13;
W34 = QP4 + W33;
WP14 = C4*WP13 + QP4*W24 + S4*WP23;
WP24 = C4*WP23 - QP4*W14 - S4*WP13;
WP34 = QDP4 + WP33;
DV14 = W14^2;
DV24 = W14*W24;
DV34 = W14*W34;
DV44 = W24^2;
DV54 = W24*W34;
DV64 = W34^2;
U114 = -DV44 - DV64;
U214 = DV24 + WP34;
U314 = DV34 - WP24;
U124 = DV24 - WP34;
U224 = -DV14 - DV64;
U324 = DV54 + WP14;
VSP14 = U113*d4 + VP13;
VSP24 = U213*d4 + VP23;
VSP34 = U313*d4 + VSP33;
VP14 = C4*VSP14 + S4*VSP24;
VP24 = C4*VSP24 - S4*VSP14;
W15 = C5*W14 - S5*W34;
W25 = -C5*W34 - S5*W14;
W35 = QP5 + W24;
WP15 = C5*WP14 + QP5*W25 - S5*WP34;
WP25 = -C5*WP34 - QP5*W15 - S5*WP14;
WP35 = QDP5 + WP24;
DV15 = W15^2;
DV25 = W15*W25;
DV35 = W15*W35;
DV45 = W25^2;
DV55 = W25*W35;
DV65 = W35^2;
U115 = -DV45 - DV65;
U215 = DV25 + WP35;
U315 = DV35 - WP25;
U125 = DV25 - WP35;
U225 = -DV15 - DV65;
U325 = DV55 + WP15;
VP15 = C5*VP14 - S5*VSP34;
VP25 = -C5*VSP34 - S5*VP14;
No31 = QDP1*ZZR1;
F32 = MXR2*U312 + MY2*U322;
PSI12 = QP2*XZR2 + W12*XXR2 + W22*XY2;
PSI22 = QP2*YZ2 + W12*XY2;
PSI32 = QP2*ZZR2 + W12*XZR2 + W22*YZ2;
No12 = -PSI22*QP2 + PSI32*W22 + QDP2*XZR2 + WP12*XXR2 + WP22*XY2;
No22 = PSI12*QP2 - PSI32*W12 + QDP2*YZ2 + WP12*XY2;
No32 = -PSI12*W22 + PSI22*W12 + QDP2*ZZR2 + WP12*XZR2 + WP22*YZ2;
F13 = MXR3*U113 + MY3*U123;
F23 = MXR3*U213 + MY3*U223;
F33 = MXR3*U313 + MY3*U323;
PSI13 = W13*XXR3 + W23*XY3 + W33*XZR3;
PSI23 = W13*XY3 + W33*YZ3;
PSI33 = W13*XZR3 + W23*YZ3 + W33*ZZR3;
No13 = -PSI23*W33 + PSI33*W23 + WP13*XXR3 + WP23*XY3 + WP33*XZR3;
No23 = PSI13*W33 - PSI33*W13 + WP13*XY3 + WP33*YZ3;
No33 = -PSI13*W23 + PSI23*W13 + WP13*XZR3 + WP23*YZ3 + WP33*ZZR3;
F14 = MX4*U114 + MYR4*U124;
F24 = MX4*U214 + MYR4*U224;
F34 = MX4*U314 + MYR4*U324;
PSI14 = W14*XXR4 + W24*XY4 + W34*XZ4;
PSI24 = W14*XY4 + W34*YZ4;
PSI34 = W14*XZ4 + W24*YZ4 + W34*ZZR4;
No14 = -PSI24*W34 + PSI34*W24 + WP14*XXR4 + WP24*XY4 + WP34*XZ4;
No24 = PSI14*W34 - PSI34*W14 + WP14*XY4 + WP34*YZ4;
No34 = -PSI14*W24 + PSI24*W14 + WP14*XZ4 + WP24*YZ4 + WP34*ZZR4;
F15 = MX5*U115 + MY5*U125;
F25 = MX5*U215 + MY5*U225;
F35 = MX5*U315 + MY5*U325;
PSI15 = W15*XXR5 + W25*XY5 + W35*XZ5;
PSI25 = W15*XY5 + W35*YZ5;
PSI35 = W15*XZ5 + W25*YZ5 + W35*ZZ5;
No15 = -PSI25*W35 + PSI35*W25 + WP15*XXR5 + WP25*XY5 + WP35*XZ5;
No25 = PSI15*W35 - PSI35*W15 + WP15*XY5 + WP35*YZ5;
No35 = -PSI15*W25 + PSI25*W15 + WP15*XZ5 + WP25*YZ5 + WP35*ZZ5;
E15 = F15 + FX5;
E25 = F25 + FY5;
E35 = F35 + FZ5;
N15 = CX5 + MY5*VP24 + No15;
N25 = CY5 - MX5*VP24 + No25;
N35 = CZ5 + MX5*VP25 - MY5*VP15 + No35;
FDI15 = C5*E15 - E25*S5;
FDI35 = -C5*E25 - E15*S5;
E14 = F14 + FDI15;
E24 = E35 + F24;
E34 = F34 + FDI35;
N14 = C5*N15 + MYR4*VSP34 - N25*S5 + No14;
N24 = -MX4*VSP34 + N35 + No24;
N34 = -C5*N25 + MX4*VP24 - MYR4*VP14 - N15*S5 + No34;
FDI14 = C4*E14 - E24*S4;
FDI24 = C4*E24 + E14*S4;
E13 = F13 + FDI14;
E23 = F23 + FDI24;
E33 = E34 + F33;
N13 = C4*N14 + MY3*VSP33 - N24*S4 + No13;
N23 = C4*N24 - E34*d4 - MXR3*VSP33 + N14*S4 + No23;
N33 = FDI24*d4 + MXR3*VP23 - MY3*VP13 + N34 + No33;
FDI23 = C3*E23 + E13*S3;
E32 = E33 + F32;
N12 = C3*N13 - MY2*VSP22 - N23*S3 + No12;
N22 = C3*N23 - E33*d3 + MXR2*VSP22 + N13*S3 + No22;
N32 = FDI23*d3 + MXR2*VP22 - MY2*VP12 + N33 + No32;
N31 = C2*N22 - E32*d2 + N12*S2 + No31;
GAM1 = FS1*sign(QP1) + FV1*QP1 + N31;
GAM2 = FS2*sign(QP2) + FV2*QP2 + N32;
GAM3 = FS3*sign(QP3) + FV3*QP3 + IA3*QDP3 + N33;
GAM4 = FS4*sign(QP4) + FV4*QP4 + IA4*QDP4 + N34;
GAM5 = FS5*sign(QP5) + FV5*QP5 + IA5*QDP5 + N35;

y = [GAM1 GAM2 GAM3 GAM4 GAM5].';

== matlab function dynmodel_KUKA/MGD_simulink ==
  data: q input; t output size=3; param parameter; R output; T output
function [t, R, T] = fcn(q,param)

th1 = q(1);
th2 = q(2);
th3 = q(3);
th4 = q(4);
th5 = q(5);

% introduction des paramètres
d1=param.d1;
r1=param.r1;
d2=param.d2;
d3=param.d3;
d4=param.d4;

% code généré OpenSymoro
C1 = cos(th1);
S1 = sin(th1);
C2 = cos(th2);
S2 = sin(th2);
T0T211 = C1*C2;
T0T221 = C2*S1;
T0T212 = -C1*S2;
T0T222 = -S1*S2;
T0T214 = C1*d2 + d1;
T0T224 = S1*d2;
C3 = cos(th3);
S3 = sin(th3);
T0T311 = C3*T0T211 + S3*T0T212;
T0T321 = C3*T0T221 + S3*T0T222;
T0T331 = C2*S3 + C3*S2;
T0T312 = C3*T0T212 - S3*T0T211;
T0T322 = C3*T0T222 - S3*T0T221;
T0T332 = C2*C3 - S2*S3;
T0T314 = T0T211*d3 + T0T214;
T0T324 = T0T221*d3 + T0T224;
T0T334 = S2*d3 + r1;
C4 = cos(th4);
S4 = sin(th4);
T0T411 = C4*T0T311 + S4*T0T312;
T0T421 = C4*T0T321 + S4*T0T322;
T0T431 = C4*T0T331 + S4*T0T332;
T0T412 = C4*T0T312 - S4*T0T311;
T0T422 = C4*T0T322 - S4*T0T321;
T0T432 = C4*T0T332 - S4*T0T331;
T0T414 = T0T311*d4 + T0T314;
T0T424 = T0T321*d4 + T0T324;
T0T434 = T0T331*d4 + T0T334;
C5 = cos(th5);
S5 = sin(th5);
T0T511 = C5*T0T411 - S1*S5;
T0T521 = C1*S5 + C5*T0T421;
T0T531 = C5*T0T431;
T0T512 = -C5*S1 - S5*T0T411;
T0T522 = C1*C5 - S5*T0T421;
T0T532 = -S5*T0T431;
T0T513 = T0T412;
T0T523 = T0T422;
T0T533 = T0T432;
T0T514 = T0T414;
T0T524 = T0T424;
T0T534 = T0T434;

R = [T0T511 T0T512 T0T513; T0T521 T0T522 T0T523; T0T531 T0T532 T0T533];
t = [T0T514 T0T524 T0T534].';
T = [R t; 0 0 0 1];

== matlab function dynmodel_KUKA/INM_simulink ==
  data: q input; dq input; Minm output size=5,5; param parameter
function Minm = fcn(q,dq, param)

th1 = q(1);
th2 = q(2);
th3 = q(3);
th4 = q(4);
th5 = q(5);

QP1 = dq(1);
QP2 = dq(2);
QP3 = dq(3);
QP4 = dq(4);
QP5 = dq(5);

% introduction des paramètres
GZ=param.GZ;
XXR2=param.XXR2;
XXR3=param.XXR3;
XXR4=param.XXR4;
XXR5=param.XXR5;
XY2=param.XY2;
XY3=param.XY3;
XY4=param.XY4;
XY5=param.XY5;
XZR2=param.XZR2;
XZR3=param.XZR3;
XZ4=param.XZ4;
XZ5=param.XZ5;
YZ2=param.YZ2;
YZ3=param.YZ3;
YZ4=param.YZ4;
YZ5=param.YZ5;
ZZR1=param.ZZR1;
ZZR2=param.ZZR2;
ZZR3=param.ZZR3;
ZZR4=param.ZZR4;
ZZ5=param.ZZ5;
MXR2=param.MXR2;
MXR3=param.MXR3;
MX4=param.MX4;
MX5=param.MX5;
MY2=param.MY2;
MY3=param.MY3;
MYR4=param.MYR4;
MY5=param.MY5;
IA3=param.IA3;
IA4=param.IA4;
IA5=param.IA5;
FV1=param.FV1;
FV2=param.FV2;
FV3=param.FV3;
FV4=param.FV4;
FV5=param.FV5;
FS1=param.FS1;
FS2=param.FS2;
FS3=param.FS3;
FS4=param.FS4;
FS5=param.FS5;
d1=param.d1;
r1=param.r1;
d2=param.d2;
d3=param.d3;
d4=param.d4;

FX5=0;
FY5=0;
FZ5=0;
CX5=0;
CY5=0;
CZ5=0;

% code généré OpenSymoro
C1 = cos(th1);
S1 = sin(th1);
C2 = cos(th2);
S2 = sin(th2);
C3 = cos(th3);
S3 = sin(th3);
C4 = cos(th4);
S4 = sin(th4);
C5 = cos(th5);
S5 = sin(th5);
AS15 = C5*MX5 - MY5*S5;
AS35 = -C5*MY5 - MX5*S5;
AJ115 = C5*XXR5 - S5*XY5;
AJ315 = -C5*XY5 - S5*XXR5;
AJ125 = C5*XY5;
AJ325 = -S5*XY5;
AJ135 = C5*XZ5 - S5*YZ5;
AJ335 = -C5*YZ5 - S5*XZ5;
AJA115 = AJ115*C5 - AJ125*S5;
AJA315 = AJ315*C5 - AJ325*S5;
AJA135 = -AJ115*S5 - AJ125*C5;
AJA335 = -AJ315*S5 - AJ325*C5;
JP114 = AJA115 + XXR4;
JP214 = AJ135 + XY4;
JP314 = AJA315 + XZ4;
JP324 = AJ335 + YZ4;
JP134 = AJA135 + XZ4;
JP334 = AJA335 + ZZR4;
MSP14 = AS15 + MX4;
AS14 = C4*MSP14 - MYR4*S4;
AS24 = C4*MYR4 + MSP14*S4;
AJ114 = C4*JP114 - JP214*S4;
AJ214 = C4*JP214 + JP114*S4;
AJ124 = C4*JP214 - S4*ZZ5;
AJ224 = C4*ZZ5 + JP214*S4;
AJ134 = C4*JP134 - JP324*S4;
AJ234 = C4*JP324 + JP134*S4;
AJA114 = AJ114*C4 - AJ124*S4;
AJA214 = AJ214*C4 - AJ224*S4;
AJA314 = C4*JP314 - JP324*S4;
AJA124 = AJ114*S4 + AJ124*C4;
AJA224 = AJ214*S4 + AJ224*C4;
AJA324 = C4*JP324 + JP314*S4;
PAS214 = AS24*d4;
PAS314 = AS35*d4;
PAS224 = -AS14*d4;
JP113 = AJA114 + XXR3;
JP213 = AJA214 - PAS214 + XY3;
JP313 = AJA314 - PAS314 + XZR3;
JP123 = AJA124 - PAS214 + XY3;
JP223 = AJA224 - 2*PAS224;
JP323 = AJA324 + YZ3;
JP133 = AJ134 - PAS314 + XZR3;
JP233 = AJ234 + YZ3;
JP333 = JP334 - 2*PAS224 + ZZR3;
MSP13 = AS14 + MXR3;
MSP23 = AS24 + MY3;
AS13 = C3*MSP13 - MSP23*S3;
AS23 = C3*MSP23 + MSP13*S3;
AJ113 = C3*JP113 - JP213*S3;
AJ213 = C3*JP213 + JP113*S3;
AJ123 = C3*JP123 - JP223*S3;
AJ223 = C3*JP223 + JP123*S3;
AJ133 = C3*JP133 - JP233*S3;
AJ233 = C3*JP233 + JP133*S3;
AJA113 = AJ113*C3 - AJ123*S3;
AJA213 = AJ213*C3 - AJ223*S3;
AJA313 = C3*JP313 - JP323*S3;
AJA123 = AJ113*S3 + AJ123*C3;
AJA223 = AJ213*S3 + AJ223*C3;
AJA323 = C3*JP323 + JP313*S3;
PAS213 = AS23*d3;
PAS313 = AS35*d3;
PAS223 = -AS13*d3;
JP112 = AJA113 + XXR2;
JP212 = AJA213 - PAS213 + XY2;
JP312 = AJA313 - PAS313 + XZR2;
JP122 = AJA123 - PAS213 + XY2;
JP222 = AJA223 - 2*PAS223;
JP322 = AJA323 + YZ2;
JP132 = AJ133 - PAS313 + XZR2;
JP232 = AJ233 + YZ2;
JP332 = JP333 - 2*PAS223 + ZZR2;
MSP12 = AS13 + MXR2;
MSP22 = AS23 + MY2;
AS12 = C2*MSP12 - MSP22*S2;
AS32 = C2*MSP22 + MSP12*S2;
AJ112 = C2*JP112 - JP212*S2;
AJ312 = C2*JP212 + JP112*S2;
AJ122 = C2*JP122 - JP222*S2;
AJ322 = C2*JP222 + JP122*S2;
AJ132 = C2*JP132 - JP232*S2;
AJ332 = C2*JP232 + JP132*S2;
AJA112 = AJ112*C2 - AJ122*S2;
AJA212 = -C2*JP312 + JP322*S2;
AJA312 = AJ312*C2 - AJ322*S2;
AJA132 = AJ112*S2 + AJ122*C2;
AJA232 = -C2*JP322 - JP312*S2;
AJA332 = AJ312*S2 + AJ322*C2;
PAS212 = -AS35*d2;
PAS312 = AS32*d2;
PAS222 = -AS12*d2;
JP211 = AJA212 - PAS212;
JP311 = AJA312 - PAS312;
JP121 = -AJ132 - PAS212;
JP221 = JP332 - 2*PAS222;
JP131 = AJA132 - PAS312;
JP331 = AJA332 - 2*PAS222 + ZZR1;
Nc21 = -C2*MSP12*d2 - JP332 + MSP22*S2*d2;
Nd32 = C3*MSP13*d3 + JP333 - MSP23*S3*d3;
Ed11 = -AS13*S2 - AS23*C2;
Ed31 = AS13*C2 - AS23*S2;
Nd11 = AJ133*C2 - AJ233*S2;
Nd21 = -AS13*C2*d2 + AS23*S2*d2 - Nd32;
Nd31 = AJ133*S2 + AJ233*C2;
Ne33 = C4*MSP14*d4 + JP334 - MYR4*S4*d4;
Ee12 = -AS14*S3 - AS24*C3;
Ee22 = AS14*C3 - AS24*S3;
Ne12 = AJ134*C3 - AJ234*S3;
Ne22 = AJ134*S3 + AJ234*C3;
Ne32 = AS14*C3*d3 - AS24*S3*d3 + Ne33;
Ee11 = C2*Ee12 - Ee22*S2;
Ee31 = C2*Ee22 + Ee12*S2;
Ne11 = C2*Ne12 - Ne22*S2;
Ne21 = -C2*Ee22*d2 - Ee12*S2*d2 - Ne32;
Ne31 = C2*Ne22 + Ne12*S2;
Ef13 = AS35*C4;
Ef23 = AS35*S4;
Nf13 = AJ135*C4 - S4*ZZ5;
Nf23 = AJ135*S4 + AS15*d4 + C4*ZZ5;
Nf33 = AJ335 + AS35*S4*d4;
Ef12 = C3*Ef13 - Ef23*S3;
Ef22 = C3*Ef23 + Ef13*S3;
Nf12 = C3*Nf13 - Nf23*S3;
Nf22 = AS15*d3 + C3*Nf23 + Nf13*S3;
Nf32 = C3*Ef23*d3 + Ef13*S3*d3 + Nf33;
Ef11 = C2*Ef12 - Ef22*S2;
Ef31 = C2*Ef22 + Ef12*S2;
Nf11 = C2*Nf12 - Nf22*S2;
Nf21 = -C2*Ef22*d2 - Ef12*S2*d2 - Nf32;
Nf31 = AS15*d2 + C2*Nf22 + Nf12*S2;
A11 = JP331;
A21 = AJ332;
A31 = Nd31;
A41 = Ne31;
A51 = Nf31;
A22 = JP332;
A32 = Nd32;
A42 = Ne32;
A52 = Nf32;
A33 = IA3 + JP333;
A43 = Ne33;
A53 = Nf33;
A44 = IA4 + JP334;
A54 = AJ335;
A55 = IA5 + ZZ5;

Minm = zeros(5);
Minm(1,1) = A11;
Minm(2,1) = A21;
Minm(3,1) = A31;
Minm(4,1) = A41;
Minm(5,1) = A51;
Minm(2,2) = A22;
Minm(3,2) = A32;
Minm(4,2) = A42;
Minm(5,2) = A52;
Minm(3,3) = A33;
Minm(4,3) = A43;
Minm(5,3) = A53;
Minm(4,4) = A44;
Minm(5,4) = A54;
Minm(5,5) = A55;

Minm = (Minm+Minm.')-diag(diag(Minm));
